simulink model "zad1v2"  (R2014b)
settings: Solver=ode45  StartTime=0.0  StopTime=70  RelTol=1e-3
undefined symbols (not defined in the file or in its folder): a1, a2, a3, a4, K, T1, T2
settings Model: Creator=kuba  LastModifiedBy=kuba

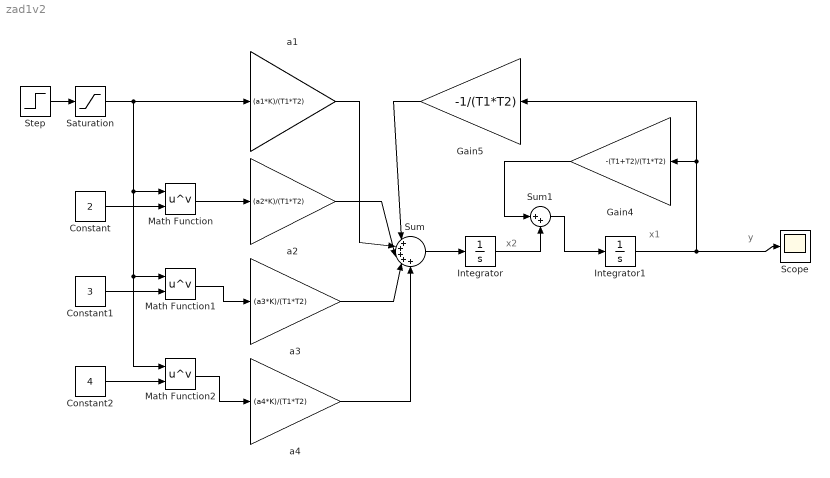
== system zad1v2 ==
  note: y
  note: x2
  note: x1
  Constant : Constant  Value=2
  Constant1 : Constant  Value=3
  Constant2 : Constant  Value=4
  Gain4 : Gain  Gain=-(T1+T2)/(T1*T2)
  Gain5 : Gain  Gain=-1/(T1*T2)
  Integrator : Integrator
  Integrator1 : Integrator
  Math Function : Math  Operator=pow  SaturateOnIntegerOverflow=on
  Math Function1 : Math  Operator=pow  SaturateOnIntegerOverflow=on
  Math Function2 : Math  Operator=pow  SaturateOnIntegerOverflow=on
  Saturation : Saturate  UpperLimit=1  LowerLimit=-1
  Scope : Scope
  Step : Step  SampleTime=0
  Sum : Sum  Inputs=|+++++
  Sum1 : Sum  Inputs=|++
  a1 : Gain  Gain=(a1*K)/(T1*T2)
  a2 : Gain  Gain=(a2*K)/(T1*T2)
  a3 : Gain  Gain=(a3*K)/(T1*T2)
  a4 : Gain  Gain=(a4*K)/(T1*T2)
  wires:
  Step/1 -> Saturation/1
  Math Function/1 -> a2/1
  Math Function1/1 -> a3/1
  Math Function2/1 -> a4/1
  a1/1 -> Sum/2
  a2/1 -> Sum/3
  a3/1 -> Sum/4
  a4/1 -> Sum/5
  Sum/1 -> Integrator/1
  Integrator/1 -> Sum1/2
  Sum1/1 -> Integrator1/1
  Integrator1/1 -> Gain5/1, Gain4/1, Scope/1
  Gain4/1 -> Sum1/1
  Gain5/1 -> Sum/1
  Constant/1 -> Math Function/2
  Constant1/1 -> Math Function1/2
  Constant2/1 -> Math Function2/2
  Saturation/1 -> Math Function2/1, Math Function1/1, Math Function/1, a1/1
